simulink library "dcl"  (Simulink 8.1)
settings: Solver=ode1  StartTime=0.0  StopTime=Inf  FixedStep=0.001  RelTol=1e-3
PostLoadFcn:
  | , if any(exist('dsrtsu_mdlpostloadfcn', 'file') == [2, 3, 6]), try dsrtsu_mdlpostloadfcn('Execute', bdroot); catch fprintf('Error in PostLoadFcn (dsrtsu_mdlpostloadfcn) for model "%s":\n %s\n', bdroot, lasterr); end, end,
libraries: pbd x1, ccb x1, pbe x1, atr x1, dcc x1, stb x1
settings Model: DSRTSU_INTERNAL_RTI_VER=450  DSRTSU_INTERNAL_RTI_TYPE=rti1401  RTICANMMDATA=struct('GeneralSetupData',struct('modelroot','D:\ELN150201_TAIWAN\trunk\AdasDragon\software\sw_development\arch\app\acc','generalsettings',struct('filesettings',struct('destfolder',struct('Name','RTICANMM_FILES','Check',1),'buildfolder',struct('Name','.','Check',1),'AbsDestfolder',struct('Name','D:\ELN150201_TAIWAN\trunk\AdasDragon\software\sw_development\arch\app\acc\RTICANMM_FILES'),'AbsBuildfolder',struct('Name','D:\ELN150201_TAIWAN\trunk\AdasDragon\software\sw_development\arch\app\acc'))),'options',struct('addpaths',1,'rmpaths',1,'addtrcexclusion',logical(1),'cannavigator',struct('checkmonitoring',0),'show_usrtrc',0,'use_usrtrc',0),'advanced',struct('options',[1 1 1 1 1 1 1 1 1 1 1 1 1 1 1 1 1 1 1 1 1 1 1 1 1 1 1 1 1 1 1 1 1 1 1 1 1 1 1 1 1 1 1 1 1 1 1 1 1 1 1 1 1 1 1 1 1 1 1 1 1 1 1 1 1 1 1 1 1 1 1 1 1 1 1 1 1 1 1 1 1 1 1 1 1 1 1 1 1 1 1 1 1 1 1 1 1 1 1 1]),'MPSetup',{{}},'modelname','dcl','block','dcl'))  DSRTSU_INTERNAL_RTIFPGA=40  Creator=tescamilla  LastModifiedBy=AT015555

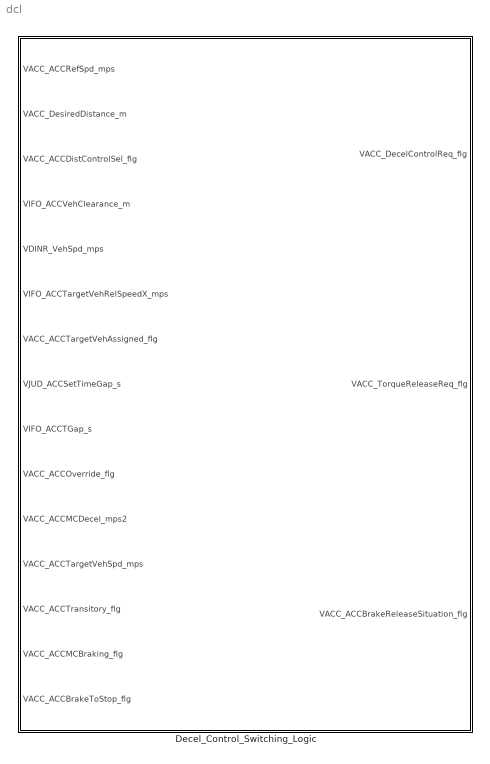
== system dcl ==
  Decel_Control_Switching_Logic : Subsystem

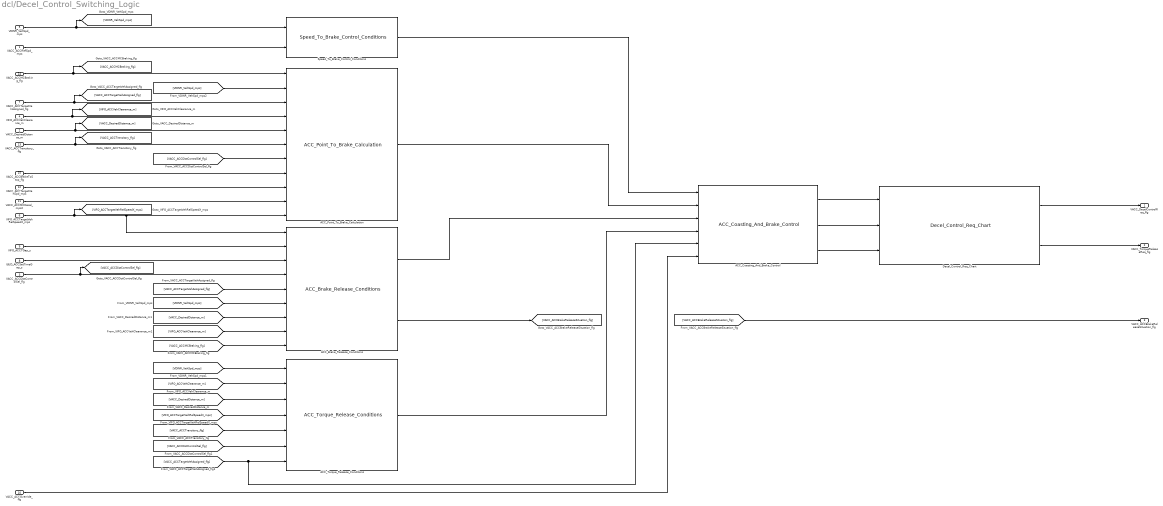
== system dcl/Decel_Control_Switching_Logic ==
  VACC_ACCRefSpd_mps : Inport
  VACC_DesiredDistance_m : Inport  Port=2
  VACC_ACCDistControlSel_flg : Inport  Port=3
  VIFO_ACCVehClearance_m : Inport  Port=4
  VDINR_VehSpd_mps : Inport  Port=5
  VIFO_ACCTargetVehRelSpeedX_mps : Inport  Port=6
  VACC_ACCTargetVehAssigned_flg : Inport  Port=7
  VJUD_ACCSetTimeGap_s : Inport  Port=8
  VIFO_ACCTGap_s : Inport  Port=9
  VACC_ACCOverride_flg : Inport  Port=10
  VACC_ACCMCDecel_mps2 : Inport  Port=11
  VACC_ACCTargetVehSpd_mps : Inport  Port=12
  VACC_ACCTransitory_flg : Inport  Port=13
  VACC_ACCMCBraking_flg : Inport  Port=14
  VACC_ACCBrakeToStop_flg : Inport  Port=15
  ACC_Brake_Release_Conditions : pbd/ACC_Brake_Release_Conditions
  ACC_Coasting_And_Brake_Control : ccb/ACC_Coasting_And_Brake_Control
  ACC_Point_To_Brake_Calculation : pbe/ACC_Point_To_Brake_Calculation
  ACC_Torque_Release_Conditions : atr/ACC_Torque_Release_Conditions
  Decel_Control_Req_Chart : dcc/Decel_Control_Req_Chart
  Speed_To_Brake_Control_Conditions : stb/Speed_To_Brake_Control_Conditions
  VACC_DecelControlReq_flg : Outport
  VACC_TorqueReleaseReq_flg : Outport  Port=2
  VACC_ACCBrakeReleaseSituation_flg : Outport  Port=3
  wires:
  VACC_DesiredDistance_m/1 -> [VACC_DesiredDistance_m], ACC_Point_To_Brake_Calculation/5
  VIFO_ACCVehClearance_m/1 -> [VIFO_ACCVehClearance_m], ACC_Point_To_Brake_Calculation/4
  VDINR_VehSpd_mps/1 -> Speed_To_Brake_Control_Conditions/1, [VDINR_VehSpd_mps]
  VACC_ACCRefSpd_mps/1 -> Speed_To_Brake_Control_Conditions/2
  Speed_To_Brake_Control_Conditions/1 -> ACC_Coasting_And_Brake_Control/1
  VIFO_ACCTargetVehRelSpeedX_mps/1 -> [VIFO_ACCTargetVehRelSpeedX_mps], ACC_Point_To_Brake_Calculation/11, ACC_Brake_Release_Conditions/1
  VIFO_ACCTGap_s/1 -> ACC_Brake_Release_Conditions/2
  VJUD_ACCSetTimeGap_s/1 -> ACC_Brake_Release_Conditions/3
  VACC_ACCTargetVehAssigned_flg/1 -> [VACC_ACCTargetVehAssigned_flg], ACC_Point_To_Brake_Calculation/3
  [VIFO_ACCVehClearance_m] -> ACC_Torque_Release_Conditions/2
  [VACC_DesiredDistance_m] -> ACC_Torque_Release_Conditions/3
  [VIFO_ACCTargetVehRelSpeedX_mps] -> ACC_Torque_Release_Conditions/4
  ACC_Point_To_Brake_Calculation/1 -> ACC_Coasting_And_Brake_Control/2
  ACC_Brake_Release_Conditions/1 -> ACC_Coasting_And_Brake_Control/3
  ACC_Torque_Release_Conditions/1 -> ACC_Coasting_And_Brake_Control/4
  Decel_Control_Req_Chart/2 -> VACC_TorqueReleaseReq_flg/1
  [VACC_ACCTargetVehAssigned_flg] -> ACC_Torque_Release_Conditions/7, ACC_Coasting_And_Brake_Control/5
  Decel_Control_Req_Chart/1 -> VACC_DecelControlReq_flg/1
  VACC_ACCOverride_flg/1 -> ACC_Coasting_And_Brake_Control/6
  ACC_Coasting_And_Brake_Control/3 -> Decel_Control_Req_Chart/3
  ACC_Coasting_And_Brake_Control/2 -> Decel_Control_Req_Chart/2
  ACC_Coasting_And_Brake_Control/1 -> Decel_Control_Req_Chart/1
  VACC_ACCDistControlSel_flg/1 -> [VACC_ACCDistControlSel_flg], ACC_Brake_Release_Conditions/4
  [VIFO_ACCVehClearance_m] -> ACC_Brake_Release_Conditions/8
  [VACC_DesiredDistance_m] -> ACC_Brake_Release_Conditions/7
  [VDINR_VehSpd_mps] -> ACC_Brake_Release_Conditions/6
  [VACC_ACCTargetVehAssigned_flg] -> ACC_Brake_Release_Conditions/5
  [VDINR_VehSpd_mps] -> ACC_Torque_Release_Conditions/1
  [VDINR_VehSpd_mps] -> ACC_Point_To_Brake_Calculation/2
  VACC_ACCTransitory_flg/1 -> [VACC_ACCTransitory_flg], ACC_Point_To_Brake_Calculation/6
  [VACC_ACCDistControlSel_flg] -> ACC_Point_To_Brake_Calculation/7
  [VACC_ACCDistControlSel_flg] -> ACC_Torque_Release_Conditions/6
  [VACC_ACCTransitory_flg] -> ACC_Torque_Release_Conditions/5
  VACC_ACCBrakeToStop_flg/1 -> ACC_Point_To_Brake_Calculation/8
  VACC_ACCTargetVehSpd_mps/1 -> ACC_Point_To_Brake_Calculation/9
  VACC_ACCMCDecel_mps2/1 -> ACC_Point_To_Brake_Calculation/10
  VACC_ACCMCBraking_flg/1 -> [VACC_ACCMCBraking_flg], ACC_Point_To_Brake_Calculation/1
  [VACC_ACCMCBraking_flg] -> ACC_Brake_Release_Conditions/9
  ACC_Brake_Release_Conditions/2 -> [VACC_ACCBrakeReleaseSituation_flg]
  [VACC_ACCBrakeReleaseSituation_flg] -> VACC_ACCBrakeReleaseSituation_flg/1
